simulink model "rtwdemo_async_local"  (R2021a)
settings: Solver=FixedStepDiscrete  StartTime=0.0  StopTime=0.5  RelTol=1e-3  AbsTol=1e-6  SampleTimeConstraint=Specified  EnableMultiTasking=on
undefined symbols (not defined in the file): DiscIntNeverNeededParam
libraries: vxlib1 x2, simulink x1
Description:
  | Asynchronous Event Modeling (VxWorks(R) OS)
  | 
  | This model shows how to simulate and generate code for asynchronous
  | events on a real-time multitasking system.
settings Model: ExtModeTrigMode=oneshot  ExtModeArmWhenConnect=off  ExtModeAutoUpdateStatusClock=off  Creator=The MathWorks, Inc.  LastModifiedBy=kvasios
settings SolverCC: AutoScaleAbsTol=off  AlgebraicLoopSolver=TrustRegion  AutoInsertRateTranBlk=on
settings DataIOCC: SaveFormat=Array  SaveOutput=off  SaveTime=off  ReturnWorkspaceOutputs=off  SignalLoggingName=sigsOut
settings OptimizationCC: DefaultParameterBehavior=Inlined  InlineInvariantSignals=on  EnhancedBackFolding=on  ExpressionDepthLimit=2147483647  StateBitsets=on  DataBitsets=on  EfficientFloat2IntCast=on  EfficientMapNaN2IntZero=off  LifeSpan=1
settings DebuggingCC: MergeDetectMultiDrivingBlocksExec=none  CheckExecutionContextPreStartOutputMsg=on  InheritedTsInSrcMsg=none  IntegerOverflowMsg=none  FcnCallInpInsideContextMsg=warning  UnconnectedInputMsg=none  UnconnectedOutputMsg=none  UnconnectedLineMsg=none  AllowSymbolicDim=off  StateNameClashWarn=warning  StrictBusMsg=ErrorOnBusTreatedAsVector  SymbolicDimsDataTypeCodeGenerationDiagnostic=none  SFUnexpectedBacktrackingDiag=warning  SFNoUnconditionalDefaultTransitionDiag=warning  SFExecutionAtInitializationDiag=none  SFMachineParentedDataDiag=warning  IntegerSaturationMsg=none  ArithmeticOperatorsInVariantConditions=warning
settings HardwareCC: TargetHWDeviceType=Generic->32-bit Embedded Processor
settings ModelReferenceCC: UpdateModelReferenceTargets=IfOutOfDate  PropagateSignalLabelsOutOfModel=off
settings SFSimCC: SimUseLocalCustomCode=off
settings RTWCC: Description=Tornado (VxWorks) Real-Time Target  SystemTargetFile=tornado.tlc  TLCOptions=-p0 -aWarnNonSaturatedBlocks=0  GenCodeOnly=on  PackageGeneratedCodeAndArtifacts=on  PackageName=rtwdemo_async_local  TemplateMakefile=tornado.tmf  GenerateReport=on  RTWVerbose=off  RTWUseLocalCustomCode=off  LaunchReport=on
settings CodeAppCC: ForceParamTrailComments=on  StateflowObjectComments=on
settings TornadoTargetCC: TargetFcnLib=ansi_tfl_tmw.mat  GenFloatMathFcnCalls=NOT IN USE  TargetLangStandard=C89/C90 (ANSI)  CodeReplacementLibrary=None  UtilityFuncGeneration=Shared location  MultiwordTypeDef=System defined  MultiwordLength=2048  DynamicStringBufferSize=256  GenerateFullHeader=on  InferredTypesCompatibility=off  GenerateSampleERTMain=off  GenerateTestInterfaces=off  ModelReferenceCompliant=off  ParMdlRefBuildCompliant=on  CompOptLevelCompliant=off  ConcurrentExecutionCompliant=off  IncludeMdlTerminateFcn=on  CombineOutputUpdateFcns=off  CombineSignalStateStructs=off  GroupInternalDataByFunction=off  SuppressErrorStatus=off  IncludeFileDelimiter=Auto  ERTCustomFileBanners=off  SupportAbsoluteTime=on  LogVarNameModifier=rt_  MatFileLogging=off  CodeInterfacePackaging=Nonreusable function  PurelyIntegerCode=off  SupportNonFinite=on  SupportComplex=on  SupportContinuousTime=on  SupportNonInlinedSFcns=on  RemoveDisableFunc=off  RemoveResetFunc=off  SupportVariableSizeSignals=off  ParenthesesLevel=Nominal  CastingMode=Nominal  MATLABClassNameForMDSCustomization=Simulink.SoftwareTarget.TargetSpecificTriggerConfigurationBase  ModelStepFunctionPrototypeControlCompliant=off  CPPClassGenCompliant=off  AutosarCompliant=off  MDXCompliant=off  GRTInterface=on  GenerateAllocFcn=off  UseToolchainInfoCompliant=off  GenerateSharedConstants=on  CoderGroups=[]  AccessMethods=[]  LookupTableObjectStructAxisOrder=1,2,3,4,...  LUTObjectStructOrderExplicitValues=Size,Breakpoints,Table  LUTObjectStructOrderEvenSpacing=Size,Breakpoints,Table  ArrayLayout=Column-major  UnsupportedSFcnMsg=error  ERTHeaderFileRootName=$R$E  ERTSourceFileRootName=$R$E  ERTDataFileRootName=$R_data  CodeFormat=RealTime  StethoScope=off  DownloadToVxWorks=off  BasePriority=30  TaskStackSize=16384  ExtMode=off  ExtModeTransport=0  ExtModeStaticAlloc=off  ExtModeStaticAllocSize=1000000  ExtModeTesting=off  ExtModeMexFile=ext_comm  ExtModeIntrfLevel=Level1  RTWCAPIParams=off  RTWCAPISignals=off
settings ConfigComp: CovMetricSettings=dw  CovSaveCumulativeToWorkspaceVar=on  CovSaveSingleToWorkspaceVar=on  CovExternalEMLEnable=off

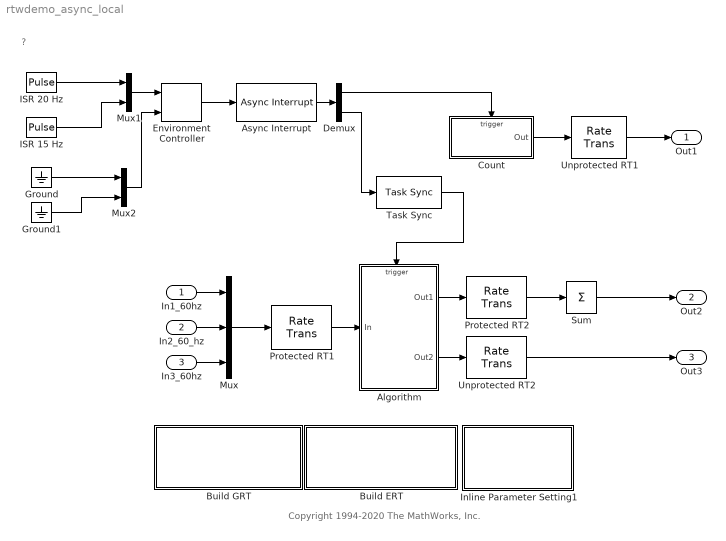
== system rtwdemo_async_local ==
  note: Copyright 1994-2020 The MathWorks, Inc.
  note: ?
  In1_60hz : Inport  OutDataTypeStr=double  PortDimensions=20  SampleTime=1/60
  In2_60_hz : Inport  Port=2  OutDataTypeStr=double  PortDimensions=20  SampleTime=1/60
  In3_60hz : Inport  Port=3  OutDataTypeStr=double  PortDimensions=20  SampleTime=1/60
  Algorithm : Subsystem  TreatAsAtomicUnit=on  RTWFcnName=Algorithm  RTWFileName=Algorithm
      settings: RTWFcnNameOpts=User specified  RTWFileNameOpts=User specified
  Async Interrupt : vxlib1/Async Interrupt  irqnumbers=[1 2]  irqoffsets=[192 193]  irqpriorities=[10 11]  irqpreempts=[0 1]  manageowntimer=on  tickres=1/60  ticklen=32bits  showinput=on
      settings: SourceProductBaseCode=SL
  Build ERT : Subsystem  mask{attrib_overrides={'IncludeMdlTerminateFcn'}}
      mask prompts: attrib_overrides "List of attributes to preserve (cell of strings):"
      mask help: Enter the attributes of the configuration set that you want preserved. Otherwise, the default configuration script will override your current settings.
      settings: OpenFcn=|
      | model=bdroot;
      |                   overrides=get_param(gcb,'attrib_overrides');
      | try
      |   rtwconfiguredemo(model,'noop',false,overrides);
      |   cs = getActiveConfigSet(bdroot);
      |   set_param(cs,'TargetOS','VxWorksExample');
      |   rtwbuilddemomodel(model);
      | catch myException
      |   rethrow(myException);
      | end
      | clear model cs overrides;
      mask Display:
      | disp(['Generate Code Using\n',...
      | 	 'Embedded Coder\n'...
      | 	  '(double-click)'])
  Build GRT : Subsystem  mask{attrib_overrides={}}
      mask prompts: attrib_overrides "List of attributes to preserve (cell of strings):"
      mask help: Enter the attributes of the configuration set that you want preserved. Otherwise, the default configuration script will override your current settings.
      settings: OpenFcn=|
      | model=bdroot;
      |                   overrides=get_param(gcb,'attrib_overrides');
      | try
      |   rtwconfiguredemo(model,'noop',true,overrides);
      |   cs = getActiveConfigSet(bdroot);
      |   cs.switchTarget('tornado.tlc',[]);
      |   set_param(cs,'TemplateMakefile','tornado.tmf');              rtwbuilddemomodel(model);
      | catch myException
      |   rethrow(myException);
      | end
      | clear model cs overrides;
      mask Display:
      | disp(['Generate Code Using\n',...
      | 	  'Simulink Coder\n',...
      | 	  '(double-click)'])
  Count : Subsystem  TreatAsAtomicUnit=on  RTWFcnName=Count  RTWFileName=Count
      settings: RTWFcnNameOpts=User specified  RTWFileNameOpts=User specified
  Demux : Demux  Outputs=2
  Environment Controller : simulink/Signal Routing/Environment Controller
      settings: SourceProductBaseCode=SL
  Ground : Ground
  Ground1 : Ground
  ISR 15 Hz : DiscretePulseGenerator  Period=4  PulseWidth=2  SampleTime=1/60
  ISR 20 Hz : DiscretePulseGenerator  Period=3  SampleTime=1/60  VectorParams1D=off
  Inline Parameter Setting1 : Subsystem
      settings: OpenFcn=m=get_param(bdroot,'name'); set_param(bdroot, 'SampleTimeColors','on'); eval([m,'([],[],[],''compile'');']); eval([m,'([],[],[],''term'');']);clear m;
      mask Display: disp(sprintf('Display Sample\nTime Colors\n(double-click)'))
  Mux : Mux  Inputs=3
  Mux1 : Mux  Inputs=2
  Mux2 : Mux  Inputs=2
  Protected RT1 : RateTransition  Deterministic=off
  Protected RT2 : RateTransition  Deterministic=off  OutPortSampleTime=1/20
  Sum : Sum  Inputs=1  InputSameDT=on  SaturateOnIntegerOverflow=on  OutDataTypeStr=Inherit: Same as first input
  Task Sync : vxlib1/Task Sync  taskname=Task0  taskpriority=50  taskstacksize=8192  parentmanaget=on  tickres=1/60  ticklen=32bits
      settings: SourceProductBaseCode=SL
  Unprotected RT1 : RateTransition  Integrity=off  OutPortSampleTime=1/20
  Unprotected RT2 : RateTransition  Integrity=off  OutPortSampleTime=1/20
  Out1 : Outport  VectorParamsAs1DForOutWhenUnconnected=off
  Out2 : Outport  Port=2  VectorParamsAs1DForOutWhenUnconnected=off
  Out3 : Outport  Port=3  VectorParamsAs1DForOutWhenUnconnected=off
  wires:
  Protected RT1/1 -> Algorithm/1(In)
  Mux/1 -> Protected RT1/1
  Algorithm/1(Out1) -> Protected RT2/1
  Protected RT2/1 -> Sum/1
  Sum/1 -> Out2/1
  Task Sync/1 -> Algorithm/Trigger
  Algorithm/2(Out2) -> Unprotected RT2/1
  Unprotected RT2/1 -> Out3/1
  Count/1(Out) -> Unprotected RT1/1
  Unprotected RT1/1 -> Out1/1
  In1_60hz/1 -> Mux/1
  In2_60_hz/1 -> Mux/2
  In3_60hz/1 -> Mux/3
  ISR 15 Hz/1 -> Mux1/2
  Environment Controller/1 -> Async Interrupt/1
  ISR 20 Hz/1 -> Mux1/1
  Mux1/1 -> Environment Controller/1
  Async Interrupt/1 -> Demux/1
  Demux/1 -> Count/Trigger
  Demux/2 -> Task Sync/1
  Ground/1 -> Mux2/1
  Ground1/1 -> Mux2/2
  Mux2/1 -> Environment Controller/2

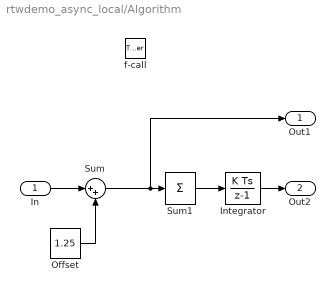
== system rtwdemo_async_local/Algorithm ==
  In : Inport
  f-call : TriggerPort  TriggerType=function-call  VariantControl=(inherit)
  Integrator : DiscreteIntegrator  SampleTime=-1  SaturateOnIntegerOverflow=on  ICPrevOutput=DiscIntNeverNeededParam  ICPrevScaledInput=DiscIntNeverNeededParam
  Offset : Constant  Value=1.25
  Sum : Sum  Inputs=|++
  Sum1 : Sum  Inputs=1  InputSameDT=on  SaturateOnIntegerOverflow=on  OutDataTypeStr=Inherit: Same as first input
  Out1 : Outport  InitialOutput=0  VectorParamsAs1DForOutWhenUnconnected=off
  Out2 : Outport  Port=2  InitialOutput=0  VectorParamsAs1DForOutWhenUnconnected=off
  wires:
  In/1 -> Sum/1
  Sum/1 -> Sum1/1, Out1/1
  Sum1/1 -> Integrator/1
  Integrator/1 -> Out2/1
  Offset/1 -> Sum/2

== system rtwdemo_async_local/Build ERT ==

== system rtwdemo_async_local/Build GRT ==

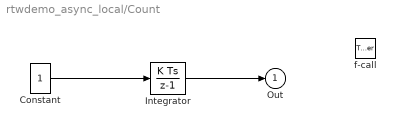
== system rtwdemo_async_local/Count ==
  f-call : TriggerPort  TriggerType=function-call  VariantControl=(inherit)
  Constant : Constant
  Integrator : DiscreteIntegrator  SampleTime=-1  SaturateOnIntegerOverflow=on  ICPrevOutput=DiscIntNeverNeededParam  ICPrevScaledInput=DiscIntNeverNeededParam
  Out : Outport  InitialOutput=0  VectorParamsAs1DForOutWhenUnconnected=off
  wires:
  Constant/1 -> Integrator/1
  Integrator/1 -> Out/1

== system rtwdemo_async_local/Inline Parameter Setting1 ==
